simulink model "buckboostconv"  (Simulink 7.5)
settings: Solver=ode45  StartTime=0.0  StopTime=.02  RelTol=1e-3
libraries: powerlib x10
settings Model: Creator=Sambhav  LastModifiedBy=Sambhav

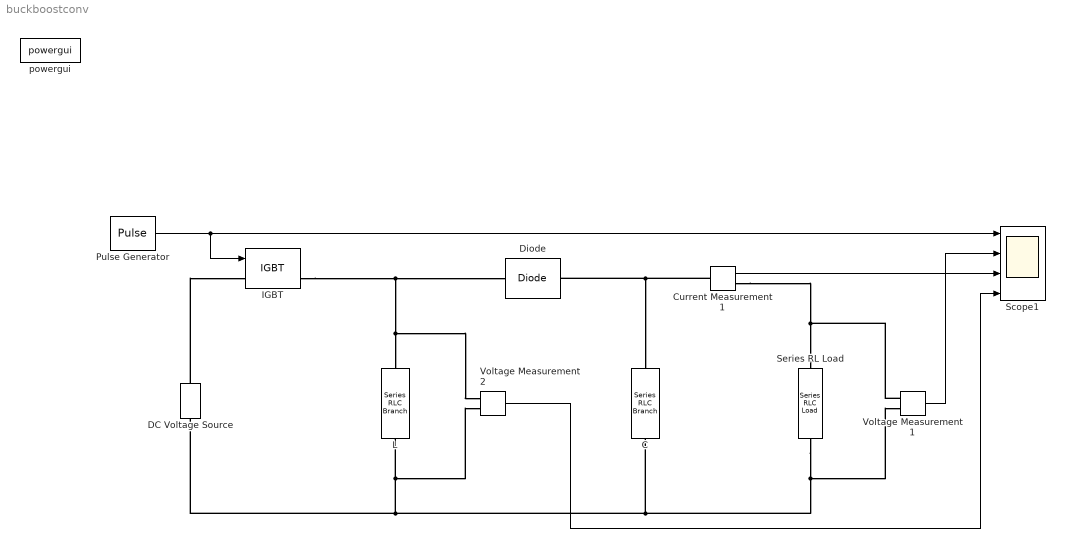
== system buckboostconv ==
  C : powerlib/Elements/Series RLC Branch  DialogController=POWERSYS.PowerSysDialog  PhysicalDomain=powersysdomain  SubClassName=unknown  LeftPortType=p1  RightPortType=p1  LConnTagsString=__new0  RConnTagsString=__new0  BranchType=C  Resistance=1  Inductance=.45e-3  SetiL0=off  InitialCurrent=0  Capacitance=10e-6  Setx0=off  InitialVoltage=0  Measurements=None
  Current Measurement1 : powerlib/Measurements/Current Measurement  DialogController=POWERSYS.PowerSysDialog  SystemSampleTime=-1  PhasorSimulation=off  OutputType=Complex  PSBequivalent=0
  DC Voltage Source : powerlib/Electrical Sources/DC Voltage Source  DialogController=POWERSYS.PowerSysDialog  SystemSampleTime=-1  Amplitude=100  Measurements=None
  Diode : powerlib/Power Electronics/Diode  DialogController=POWERSYS.PowerSysDialog  SystemSampleTime=-1  Ron=0.001  Lon=0  Vf=0.8  IC=0  UseSnubber=off  Rs=500  Cs=250e-9  Measurements=off
  IGBT : powerlib/Power Electronics/IGBT  DialogController=POWERSYS.PowerSysDialog  SystemSampleTime=-1  Ron=0.001  Lon=0  Vf=1  Tf=1e-6  Tt=2e-6  IC=0  Rs=1e5  Cs=inf  Measurements=on
  L : powerlib/Elements/Series RLC Branch  DialogController=POWERSYS.PowerSysDialog  PhysicalDomain=powersysdomain  SubClassName=unknown  LeftPortType=p1  RightPortType=p1  LConnTagsString=__new0  RConnTagsString=__new0  BranchType=L  Resistance=1  Inductance=.45e-3  SetiL0=off  InitialCurrent=0  Capacitance=1e-6  Setx0=off  InitialVoltage=0  Measurements=None
  Pulse Generator : DiscretePulseGenerator  PulseType=Time based  Amplitude=1  Period=1/25000  PulseWidth=20  PhaseDelay=0  SampleTime=1
  Scope1 : Scope  NumInputPorts=4
      settings: TimeRange=0.02  YMin=0~-600~-6~-5  YMax=1.2~100~1~5
  Series RL Load : powerlib/Elements/Series RLC Load  DialogController=POWERSYS.PowerSysDialog  PhysicalDomain=powersysdomain  SubClassName=unknown  LeftPortType=p1  RightPortType=p1  LConnTagsString=a  RConnTagsString=__new0  NominalVoltage=100  NominalFrequency=25000  ActivePower=100  InductivePower=100  CapacitivePower=0  Setx0=off  InitialVoltage=0  SetiL0=off  InitialCurrent=0  Measurements=None
  Voltage Measurement1 : powerlib/Measurements/Voltage Measurement  DialogController=POWERSYS.PowerSysDialog  SystemSampleTime=-1  PhasorSimulation=off  OutputType=Complex  PSBequivalent=0
  Voltage Measurement2 : powerlib/Measurements/Voltage Measurement  DialogController=POWERSYS.PowerSysDialog  SystemSampleTime=-1  PhasorSimulation=off  OutputType=Complex  PSBequivalent=0
  powergui : powerlib/powergui  SystemSampleTime=-1  SimulationMode=Continuous  SampleTime=50e-6  frequency=60  SPID=off  DisableSnubberDevices=off  DisableRonSwitches=off  DisableVfSwitches=off  SwTol=0  Interpol=off  frequencyindice=0  echomessages=off  HookPort=off  DisplayEquations=off  FunctionMessages=off  EnableUseOfTLC=off  x0status=blocks  RestoreLinks=warning  ResistiveCurrentMeasurement=off  Frange=[0:2:500]  Ylog=off  Xlog=on  ShowGrid=off  save=off  variable=ZData  ZoomFFT=on  StartTime=0.0  cycles=1  DisplayStyle=1  fundamental=60  FreqAxis=off  MaxFrequency=1000  frequencyindicesteady=1  RmsSteady=1  display=off  Ts=0  methode=off
  wires:
  Pulse Generator/1 -> IGBT/1, Scope1/1
  Voltage Measurement1/1 -> Scope1/2
  Current Measurement1/1 -> Scope1/3
  Voltage Measurement2/1 -> Scope1/4
  connections:
  DC Voltage Source/RConn1 -- IGBT/LConn1
  IGBT/RConn1 -- Diode/RConn1 -- L/RConn1 -- Voltage Measurement2/LConn1
  Voltage Measurement1/LConn1 -- Series RL Load/LConn1 -- Current Measurement1/RConn1
  DC Voltage Source/LConn1 -- Series RL Load/RConn1 -- Voltage Measurement1/LConn2 -- C/LConn1 -- L/LConn1 -- Voltage Measurement2/LConn2
  Current Measurement1/LConn1 -- Diode/LConn1 -- C/RConn1
